simulink model "math_reciprocal"  (Simulink 6.3)
settings: Solver=FixedStepDiscrete  StartTime=0.0  StopTime=10.0  FixedStep=1  RelTol=1e-3
settings Model: Creator=ksmyth  LastModifiedBy=hnine
settings DebuggingCC: SignalResolutionControl=UseLocalSettings  MultiTaskDSMMsg=error

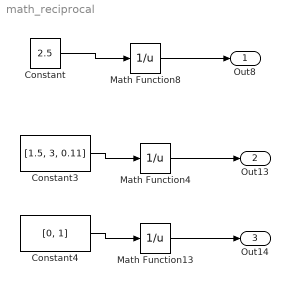
== system math_reciprocal ==
  Constant : Constant  Value=2.5
  Constant3 : Constant  Value=[1.5, 3, 0.11]
  Constant4 : Constant  Value=[0, 1]
  Math Function13 : Math  Operator=reciprocal  SaturateOnIntegerOverflow=on
  Math Function4 : Math  Operator=reciprocal  SaturateOnIntegerOverflow=on
  Math Function8 : Math  Operator=reciprocal  SaturateOnIntegerOverflow=on
  Out8 : Outport
  Out13 : Outport  Port=2
  Out14 : Outport  Port=3
  wires:
  Constant/1 -> Math Function8/1
  Math Function8/1 -> Out8/1
  Constant3/1 -> Math Function4/1
  Math Function4/1 -> Out13/1
  Constant4/1 -> Math Function13/1
  Math Function13/1 -> Out14/1
